simulink model "auto4exp"  (Simulink 8.2)
settings: Solver=ode4  StartTime=0.0  StopTime=10.0  RelTol=1e-3
libraries: simulink x1
settings Model: Creator=nathanlrf  LastModifiedBy=nathanlrf
settings DataIOCC: SignalLoggingSaveFormat=Dataset
settings OptimizationCC: ExpressionDepthLimit=128
settings DebuggingCC: FcnCallInpInsideContextMsg=EnableAllAsError  StateNameClashWarn=none
settings GRTTargetCC: CombineOutputUpdateFcns=on  GRTInterface=off

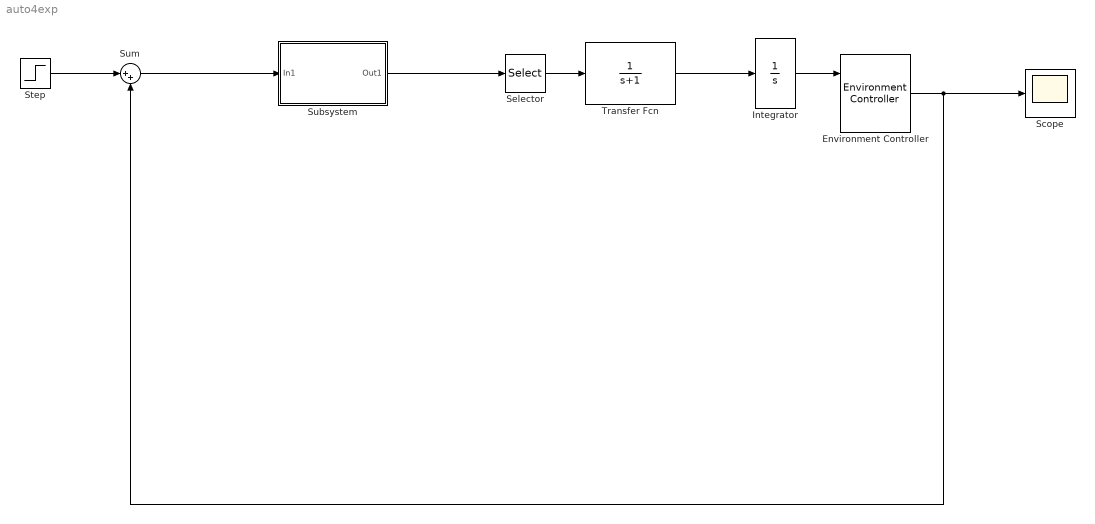
== system auto4exp ==
  Environment Controller : simulink/Signal Routing/Environment Controller
  Integrator : Integrator
  Scope : Scope
  Selector : Selector  InputPortWidth=4  IndexOptions=Index vector (dialog)  Indices=2  OutputSizes=1
  Step : Step  SampleTime=0
  Subsystem : Subsystem
  Sum : Sum  Inputs=|++
  Transfer Fcn : TransferFcn  Denominator=[1 1]
  wires:
  Step/1 -> Sum/1
  Selector/1 -> Transfer Fcn/1
  Transfer Fcn/1 -> Integrator/1
  Integrator/1 -> Environment Controller/1
  Environment Controller/1 -> Scope/1, Sum/2
  Subsystem/1(Out1) -> Selector/1
  Sum/1 -> Subsystem/1(In1)

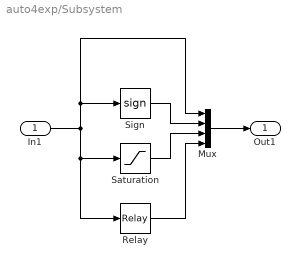
== system auto4exp/Subsystem ==
  In1 : Inport
  Mux : Mux
  Relay : Relay  OnSwitchValue=0.5  OffSwitchValue=-0.5  OffOutputValue=-1
  Saturation : Saturate
  Sign : Signum
  Out1 : Outport
  wires:
  Relay/1 -> Mux/4
  Saturation/1 -> Mux/3
  In1/1 -> Mux/1, Sign/1, Saturation/1, Relay/1
  Sign/1 -> Mux/2
  Mux/1 -> Out1/1
